simulink model "sim_cs3_2"  (R2022b)
settings: Solver=ode4  StartTime=0.0  StopTime=10.0  FixedStep=tstep  RelTol=1e-3
undefined symbols (not defined in the file): K
settings Model: Creator=dipte  LastModifiedBy=dipte
settings DataIOCC: ReturnWorkspaceOutputs=off

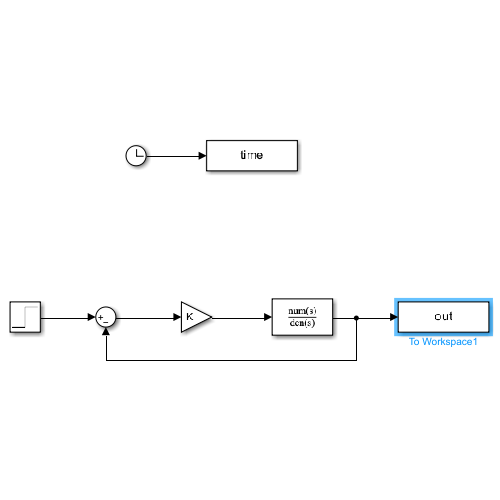
[thumbnail: Simulink's stored preview of the top-level diagram]
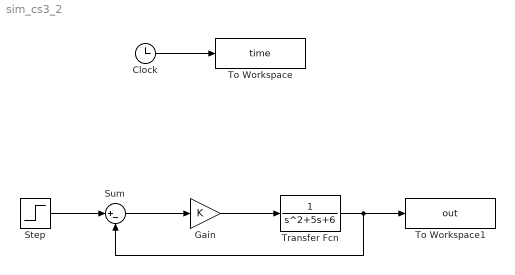
== system sim_cs3_2 ==
  Clock : Clock
  Gain : Gain  Gain=K
  Step : Step  SampleTime=0
  Sum : Sum  Inputs=|+-
  To Workspace : ToWorkspace  VariableName=time  SampleTime=-1
      settings: Save2DSignal=2-D array (concatenate along first dimension)
  To Workspace1 : ToWorkspace  VariableName=out  SampleTime=-1
      settings: Save2DSignal=2-D array (concatenate along first dimension)
  Transfer Fcn : TransferFcn  Denominator=[1 5 6]
  wires:
  Step/1 -> Sum/1
  Sum/1 -> Gain/1
  Gain/1 -> Transfer Fcn/1
  Transfer Fcn/1 -> Sum/2, To Workspace1/1
  Clock/1 -> To Workspace/1
